simulink model "motor_sim"  (R2019b)
settings: Solver=ode5  StartTime=0.0  StopTime=t_s  FixedStep=h  RelTol=1e-3  EnableMultiTasking=on
undefined symbols (not defined in the file): A, B
settings Model: Creator=erdem  LastModifiedBy=Claudia Yasar
settings DataIOCC: LimitDataPoints=on  ReturnWorkspaceOutputs=off
settings OptimizationCC: LifeSpan=inf
settings DebuggingCC: AllowSymbolicDim=off  SFUnexpectedBacktrackingDiag=warning  SFNoUnconditionalDefaultTransitionDiag=warning  SFExecutionAtInitializationDiag=none  ArithmeticOperatorsInVariantConditions=warning
settings ModelReferenceCC: PropagateSignalLabelsOutOfModel=off
settings SFSimCC: SimUseLocalCustomCode=off  CustomCodeUndefinedFunction=UseInterfaceOnly
settings RTWCC: RTWUseLocalCustomCode=off
settings CodeAppCC: StateflowObjectComments=on
settings GRTTargetCC: TargetLangStandard=C89/C90 (ANSI)
settings ConfigComp: CovMetricSettings=dw  CovHtmlReporting=on  CovSaveCumulativeToWorkspaceVar=on  CovSaveSingleToWorkspaceVar=on  CovExternalEMLEnable=off

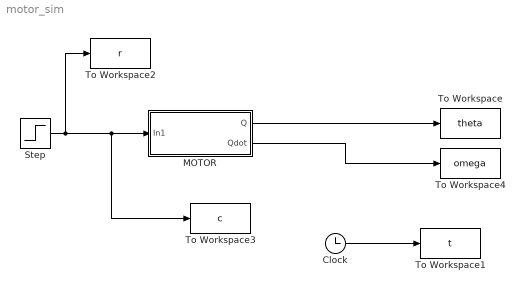
== system motor_sim ==
  Clock : Clock
  MOTOR : Subsystem
  Step : Step  SampleTime=0
  To Workspace : ToWorkspace  VariableName=theta  SampleTime=-1
  To Workspace1 : ToWorkspace  VariableName=t  SampleTime=-1
  To Workspace2 : ToWorkspace  VariableName=r  SampleTime=-1
  To Workspace3 : ToWorkspace  VariableName=c  SampleTime=-1
  To Workspace4 : ToWorkspace  VariableName=omega  SampleTime=-1
  wires:
  Step/1 -> To Workspace3/1, MOTOR/1(In1), To Workspace2/1
  MOTOR/1(Q) -> To Workspace/1
  Clock/1 -> To Workspace1/1
  MOTOR/2(Qdot) -> To Workspace4/1

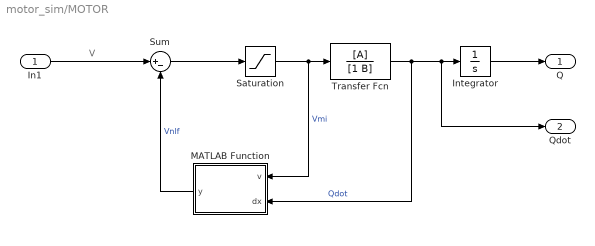
== system motor_sim/MOTOR ==
  note: V
  In1 : Inport
  Integrator : Integrator
  MATLAB Function : MATLAB Function  TreatAsAtomicUnit=on
  Saturation : Saturate  UpperLimit=1  LowerLimit=-1
  Sum : Sum  Inputs=|+-
  Transfer Fcn : TransferFcn  Numerator=[A]  Denominator=[1 B]
  Q : Outport
  Qdot : Outport  Port=2
  wires:
  Transfer Fcn/1 -> MATLAB Function/2(dx), Qdot/1, Integrator/1  "Qdot"
  Saturation/1 -> MATLAB Function/1(v), Transfer Fcn/1  "Vmi"
  Integrator/1 -> Q/1
  In1/1 -> Sum/1
  Sum/1 -> Saturation/1
  MATLAB Function/1(y) -> Sum/2  "Vnlf"

== matlab function motor_sim/MOTOR/MATLAB Function ==
  data: v input; y output; dx input
function y = fcn(v, dx)
%#codegen
Vie=0.15;
if dx==0
    if abs(v)<=Vie
        y=v;
    else 
        y=sign(v)*Vie;
    end
else
    y=Vie*sign(dx);
end
